simulink model "un_110dB_DTDSM_1b_2or_1024osr"  (R2019b)
settings: Solver=VariableStepAuto  StartTime=0.0  StopTime=ts*(Mpoints+10)  RelTol=1e-3
InitFcn:
  | %fs=256*2e4;
  | %osr=512;
  | ts=1/fs;
  | 
  | Ncycle=21;
  | Mpoints=2^16;
  | fin=fs*Ncycle/Mpoints;
  | 
  | 
  | ref=2;
values from neighbouring files (symbols this model uses):
  fs = osr*2*2e4    (= 40960000)    [CTSDM.m]
  osr = 1024    [CTSDM.m]    (also in ENOB.m = logspace(log10(64), log10(2^15), 1000); SNR.m = logspace(log10(64), log10(2^15), 1000))
undefined symbols (not defined in the file or in its folder): argo
libraries: SDtoolbox x4
settings Model: Creator=lenovo  LastModifiedBy=lenovo

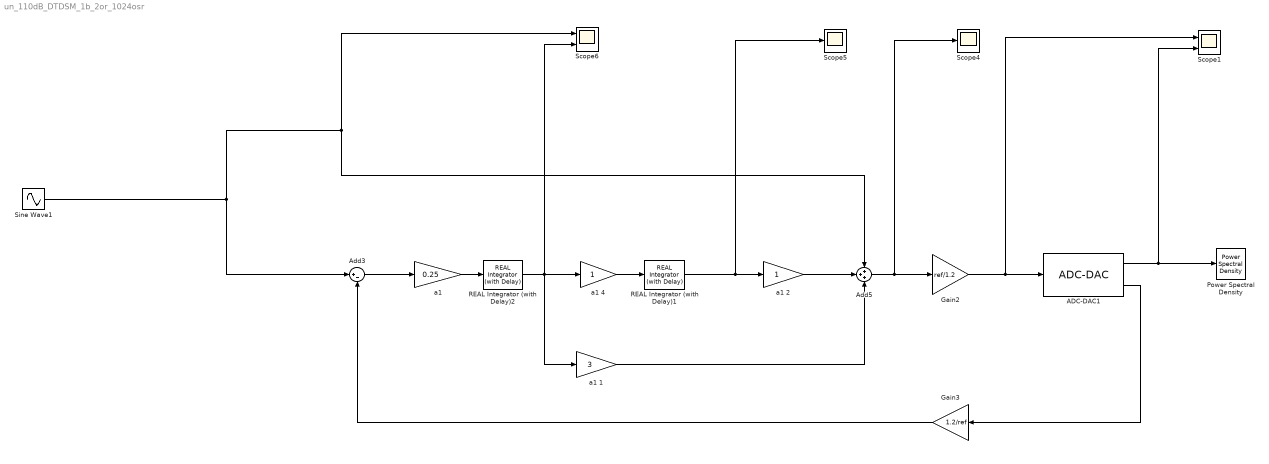
== system un_110dB_DTDSM_1b_2or_1024osr ==
  ADC-DAC1 : SDtoolbox/ADC-DAC  k=1  MM=off  match=0  CST=0  VVG=off  argo=argo(:,3)  LF=on  NF=retA.log
      settings: SourceProductName=SDtoolbox
  Add3 : Sum  Inputs=|+-
  Add5 : Sum  Inputs=+++
  Gain2 : Gain  Gain=ref/1.2
  Gain3 : Gain  Gain=1.2/ref
  Power Spectral Density : SDtoolbox/Power Spectral Density  SN=2  Fs=fs  fBL=1  fBH=fs/(2*osr)  Fin=fin  N=Mpoints  Ntransient=10  VW=on  savename=20  Scale_type=logarithmic
      settings: SourceProductName=SDtoolbox
  REAL Integrator (with Delay)1 : SDtoolbox/REAL Integrator (with Delay)  Ts=ts  alfa=(1e4-1)/1e4  Amax=1  sr=1e7  GBW=1e8
      settings: SourceProductName=SDtoolbox
  REAL Integrator (with Delay)2 : SDtoolbox/REAL Integrator (with Delay)  Ts=ts  alfa=(1e4-1)/1e4  Amax=A  sr=1E8  GBW=1E7
      settings: SourceProductName=SDtoolbox
  Scope1 : Scope  NumInputPorts=2
  Scope4 : Scope
  Scope5 : Scope
  Scope6 : Scope  NumInputPorts=2
  Sine Wave1 : Sin  Amplitude=0.5  Frequency=fin*2*pi  SampleTime=ts
  "a1 " : Gain  Gain=0.25
  a1 1 : Gain  Gain=3
  a1 2 : Gain
  a1 4 : Gain
  wires:
  Add5/1 -> Scope4/1, Gain2/1
  Add3/1 -> "a1 "/1
  REAL Integrator (with Delay)2/1 -> Scope6/2, a1 1/1, a1 4/1
  a1 4/1 -> REAL Integrator (with Delay)1/1
  ADC-DAC1/1 -> Scope1/2, Power Spectral Density/1
  a1 1/1 -> Add5/3
  REAL Integrator (with Delay)1/1 -> a1 2/1, Scope5/1
  Gain3/1 -> Add3/2
  a1 2/1 -> Add5/2
  ADC-DAC1/2 -> Gain3/1
  "a1 "/1 -> REAL Integrator (with Delay)2/1
  Gain2/1 -> Scope1/1, ADC-DAC1/1
  Sine Wave1/1 -> Add3/1, Add5/1, Scope6/1
